simulink model "ex15"  (R2023b)
settings: Solver=FixedStepDiscrete  StartTime=0.0  StopTime=200.0  FixedStep=1  RelTol=1e-3
Description:
  | Fixed-Point Direct Form Filter
  | 
  | This example shows how to implement a direct form filter in fixed point
  | using fundamental building blocks such as Gain, Delay, and Sum.
settings Model: MinMaxOverflowLogging=MinMaxAndOverflow  Creator=The MathWorks, Inc.  LastModifiedBy=eechris
settings SolverCC: AlgebraicLoopSolver=TrustRegion  MaxZcPerStep=1
settings DataIOCC: SaveFormat=Array  ReturnWorkspaceOutputs=off  SignalLoggingName=sigsOut
settings OptimizationCC: BooleanDataType=off  ExpressionDepthLimit=2147483647  InitFltsAndDblsToZero=on  LifeSpan=inf
settings DebuggingCC: SaveWithParameterizedLinksMsg=none  UnderspecifiedInitializationDetection=Classic  MergeDetectMultiDrivingBlocksExec=none  SignalResolutionControl=TryResolveAllWithWarning  MultiTaskDSMMsg=warning  MultiTaskCondExecSysMsg=none  IntegerOverflowMsg=none  ParameterDowncastMsg=warning  ParameterOverflowMsg=warning  ParameterPrecisionLossMsg=none  FcnCallInpInsideContextMsg=warning  UnconnectedInputMsg=warning  UnconnectedOutputMsg=warning  UnconnectedLineMsg=warning  StateNameClashWarn=warning  SFUnexpectedBacktrackingDiag=warning  SFNoUnconditionalDefaultTransitionDiag=warning  SFExecutionAtInitializationDiag=none  IntegerSaturationMsg=none  ArithmeticOperatorsInVariantConditions=warning
settings HardwareCC: ProdBitPerPointer=32  ProdBitPerSizeT=32  ProdBitPerPtrDiffT=32  ProdLargestAtomicFloat=None  ProdIntDivRoundTo=Undefined  ProdEndianess=Unspecified  ProdWordSize=32  ProdHWDeviceType=32-bit Generic  TargetUnknown=on
settings ModelReferenceCC: EnableRefExpFcnMdlSchedulingChecks=on  PropagateSignalLabelsOutOfModel=off
settings SFSimCC: SimUseLocalCustomCode=off  CustomCodeUndefinedFunction=UseInterfaceOnly
settings RTWCC: RTWUseLocalCustomCode=off  DLArmComputeVersion=19.05
settings CodeAppCC: StateflowObjectComments=on
settings GRTTargetCC: TargetFcnLib=ansi_tfl_tmw.mat  TargetLangStandard=C89/C90 (ANSI)  CombineOutputUpdateFcns=off  GRTInterface=on
settings ConfigComp: CovMetricSettings=d  CovSaveCumulativeToWorkspaceVar=on  CovSaveSingleToWorkspaceVar=on  CovExternalEMLEnable=off

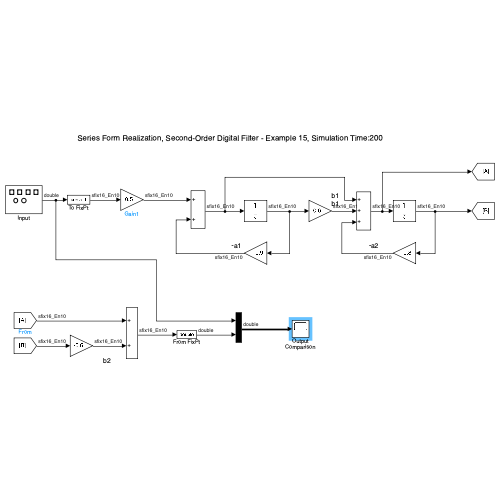
[thumbnail: Simulink's stored preview of the top-level diagram]
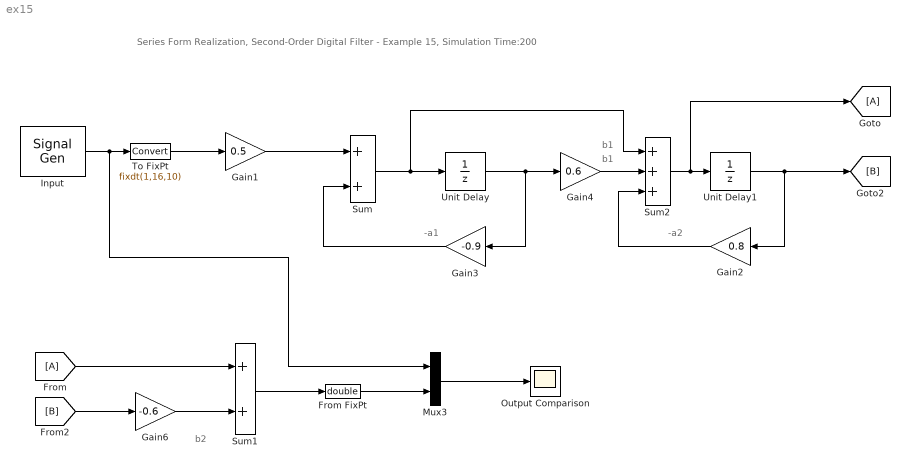
== system ex15 ==
  note: b1
  note: -a2
  note: Series Form Realization, Second-Order Digital Filter - Example 15, Simulation Time:200
  note: -a1
  note: b2
  note: b1
  From : From
  From FixPt : DataTypeConversion  OutDataTypeStr=double  SaturateOnIntegerOverflow=off  RndMeth=Floor
  Gain1 : Gain  Gain=0.5  ParamDataTypeStr=sfix( 16 )  OutDataTypeStr=fixdt(1,16,10)
  Gain2 : Gain  Gain=0.8  ParamDataTypeStr=sfix( 16 )  OutDataTypeStr=fixdt(1,16,10)
  Gain3 : Gain  Gain=-0.9  ParamDataTypeStr=sfix( 16 )  OutDataTypeStr=fixdt(1,16,10)
  Gain4 : Gain  Gain=0.6  ParamDataTypeStr=sfix( 16 )  OutDataTypeStr=fixdt(1,16,10)
  Gain6 : Gain  Gain=-0.6  ParamDataTypeStr=sfix( 16 )  OutDataTypeStr=fixdt(1,16,10)
  Goto : Goto
  Input : SignalGenerator  WaveForm=square  Frequency=0.005
  Mux3 : Mux  Inputs=2
  Output Comparison : Scope
  Sum : Sum  OutDataTypeStr=fixdt(1,16,10)
  Sum1 : Sum  OutDataTypeStr=fixdt(1,16,10)
  Sum2 : Sum  Inputs=+++  OutDataTypeStr=fixdt(1,16,10)
  To FixPt : DataTypeConversion  OutDataTypeStr=fixdt(1,16,10)  SaturateOnIntegerOverflow=off  RndMeth=Floor
  Unit Delay : UnitDelay  InitialCondition=0.0  SampleTime=1.0  HasFrameUpgradeWarning=on
  Unit Delay1 : UnitDelay  InitialCondition=0.0  SampleTime=1.0  HasFrameUpgradeWarning=on
  wires:
  Sum/1 -> Unit Delay/1, Sum2/1
  Unit Delay/1 -> Gain4/1, Gain3/1
  Unit Delay1/1 -> [B], Gain2/1
  Sum1/1 -> From FixPt/1
  From FixPt/1 -> Mux3/2
  Mux3/1 -> Output Comparison/1
  From/1 -> Sum1/1
  Gain3/1 -> Sum/2
  Gain4/1 -> Sum2/2
  Gain2/1 -> Sum2/3
  Sum2/1 -> Goto/1, Unit Delay1/1
  [B] -> Gain6/1
  Gain6/1 -> Sum1/2
  Input/1 -> Mux3/1, To FixPt/1
  Gain1/1 -> Sum/1
  To FixPt/1 -> Gain1/1
